simulink model "Islanding_case"  (R2024b)
settings: Solver=ode3  StartTime=0.0  StopTime=2.8  FixedStep=Ts  RelTol=1e-3  EnableMultiTasking=on
InitFcn:
  | Ts=100e-6;
  | Ts_Control=100e-6;
  | Ts_Power=100e-6;
  | tvv=0.1;
  | tr=1;
  | RelayEnableTime=1;
  | En_MC=1;
  | 
  | % ================= CHOOSE THE CASE HERE ==================
  | CaseNo    = 1;      % 1 = grid connected   2 = islanding   3 = fault during islanding
  | FaultType = 'none';   % 'none'  'LG'  'LL'  'LLG'  'LLL'  'LLLG'   (not used in case 2)
  | Qmismatch = 0;      % extra capacitive reactive power (% of 1.5 MW per load); try 1 in case 2 to see the inverter trip
  | % =========================================================
  | 
  | % ---- settings derived from the case (no need to edit)
  | switch CaseNo
  |     case 1, Tisland = 100; Pmismatch = 50; Tf = 2.0;   % grid + PV supply the load, fault at 2.0 s
  |     case 2, Tisland = 2.0; Pmismatch = 0;  Tf = 100;   % breakers open at 2.0 s, no fault
  |     case 3, Tisland = 2.0; Pmismatch = 0;  Tf = 2.3;   % breakers open at 2.0 s, fault at 2.3 s
  |     otherwise, error('CaseNo must be 1, 2 or 3');
  | end
  | FaultDur = 0.1;     % fault duration (s)
  | Tf_LG   = 100; Tf_LL = 100; Tf_LLG = 100; Tf_LLL = 100; Tf_LLLG = 100;   % 100 = never
  | switch upper(FaultType)
  |     case 'LG',   Tf_LG   = Tf;
  |     case 'LL',   Tf_LL   = Tf;
  |     case 'LLG',  Tf_LLG  = Tf;
  |     case 'LLL',  Tf_LLL  = Tf;
  |     case 'LLLG', Tf_LLLG = Tf;
  |     case 'NONE'
  |     otherwise, error('FaultType must be none, LG, LL, LLG, LLL or LLLG');
  | end
undefined symbols (not defined in the file or in its folder): DiscIntNeverNeededParam, Finit, Newton, Raphson, Tisland
libraries: simulink x33, spsOnDelayLib x17, powerlib_extras x11, eeGeneralControl x9, spsThreePhaseFaultLib x6, slpidlib x6, spsThreePhaseVIMeasurementLib x4, spsSampleandHoldLib x4, spsAlphaBetaZerotodq0Lib x4, spsThreePhaseSourceLib x4, spsThreePhaseBreakerLib x3, simulink_extras x3
(part 2 of 4)

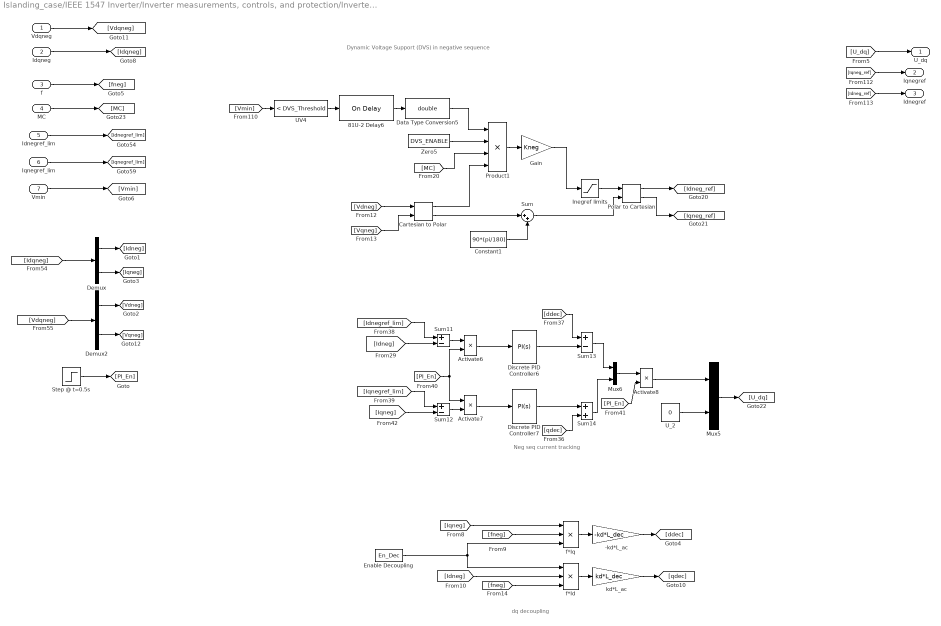
== system Islanding_case/IEEE 1547 Inverter/Inverter measurements, controls, and protection/Inverter control in negative sequence ==
  note: dq decoupling
  note: Neg seq current tracking
  note: Dynamic Voltage Support (DVS) in negative sequence
  Vdqneg : Inport
  Idqneg : Inport  Port=2
  f : Inport  Port=3
  MC : Inport  Port=4
  Idnegref_lim : Inport  Port=5
  Iqnegref_lim : Inport  Port=6
  Vmin : Inport  Port=7
  -kd*L_ac : Gain  Gain=-kd*L_dec  SaturateOnIntegerOverflow=on  OutDataTypeStr=Inherit: Same as input  ParamDataTypeStr=Inherit: Same as input
  81U-2 Delay6 : spsOnDelayLib/On Delay  DelayType=Off delay  delay=0.016  ic=0  Ts=0
  Activate6 : Product  OutDataTypeStr=double  RndMeth=Zero
  Activate7 : Product  OutDataTypeStr=double  RndMeth=Zero
  Activate8 : Product  OutDataTypeStr=double  RndMeth=Zero
  Cartesian to Polar : simulink_extras/Transformations/Cartesian to Polar
  Constant1 : Constant  Value=90*(pi/180)
  Data Type Conversion5 : DataTypeConversion  OutDataTypeStr=double  SaturateOnIntegerOverflow=off  RndMeth=Floor
  Demux : Demux  Outputs=2
  Demux2 : Demux  Outputs=2
  Discrete PID Controller6 : slpidlib/PID Controller  Controller=PI  Form=Parallel  TimeDomain=Continuous-time  UseExternalTs=off  SampleTime=-1  IntegratorMethod=Forward Euler  FilterMethod=Forward Euler  ControllerParametersSource=internal  P=Kpi  I=Kii  UseKiTs=off  D=0  UseExternalDerivativeSource=off  N=100  UseFilter=on  TunerSelectOption=Transfer Function Based (PID Tuner App)  InitialConditionSource=internal  InitialConditionForIntegrator=0  InitialConditionForFilter=0  DifferentiatorICPrevScaledInput=0  ExternalReset=none  TrackingMode=off  Kt=1  LimitOutput=on  SatLimitsSource=internal  UpperSaturationLimit=1  LowerSaturationLimit=-1  LinearizeAsGain=off  AntiWindupMode=none  Kb=1  LimitIntegrator=off  UpperIntegratorSaturationLimit=inf  LowerIntegratorSaturationLimit=-inf  POutMin=[]  POutMax=[]  IOutMin=[]  IOutMax=[]  DOutMin=[]  DOutMax=[]  NOutMin=[]  NOutMax=[]  SumOutMin=[]  SumOutMax=[]  SaturationOutMin=[]  SaturationOutMax=[]  PParamMin=[]  PParamMax=[]  IParamMin=[]  IParamMax=[]  DParamMin=[]  DParamMax=[]  NParamMin=[]  NParamMax=[]  KbParamMin=[]  KbParamMax=[]  KtParamMin=[]  KtParamMax=[]  KbOutMin=[]  KbOutMax=[]  KtOutMin=[]  KtOutMax=[]  IntegratorOutMin=[]  IntegratorOutMax=[]  FilterOutMin=[]  FilterOutMax=[]  SumI1OutMin=[]  SumI1OutMax=[]  SumI2OutMin=[]  SumI2OutMax=[]  SumI3OutMin=[]  SumI3OutMax=[]  SumI4OutMin=[]  SumI4OutMax=[]  SumDOutMin=[]  SumDOutMax=[]  DifferentiatorOutMin=[]  DifferentiatorOutMax=[]  FilterDiffOutCoefMin=[]  FilterDiffOutCoefMax=[]  ReciprocalOutMin=[]  ReciprocalOutMax=[]  SumDenOutMin=[]  SumDenOutMax=[]  SumNumOutMin=[]  SumNumOutMax=[]  DivideOutMin=[]  DivideOutMax=[]  UdiffTsProdOutMin=[]  UdiffTsProdOutMax=[]  NTsProdOutMin=[]  NTsProdOutMax=[]  UintegralTsProdOutMin=[]  UintegralTsProdOutMax=[]  UngainTsProdOutMin=[]  UngainTsProdOutMax=[]  ClampingZeroOutDataTypeStr=Inherit: Inherit via back propagation  ClampingZeroOutMin=[]  ClampingZeroOutMax=[]  FilterDenConstantOutDataTypeStr=Inherit: Inherit via back propagation  FilterDenConstantOutMin=[]  FilterDenConstantOutMax=[]  PCopyOutDataTypeStr=Inherit: Inherit via back propagation  PCopyOutMin=[]  PCopyOutMax=[]  NCopyOutDataTypeStr=Inherit: Inherit via back propagation  NCopyOutMin=[]  NCopyOutMax=[]  IntegratorContinuousStateAttributes=''  IntegratorStateMustResolveToSignalObject=off  IntegratorRTWStateStorageClass=Auto  FilterContinuousStateAttributes=''  FilterStateMustResolveToSignalObject=off  FilterRTWStateStorageClass=Auto  ParallelPVariant=InternalParameters  IdealPVariant=Disabled  IVariant=InternalParameters  DVariant=Disabled  IntegratorVariant=Continuous  SatVariant=Enabled  AWVariant=Passthrough  PCopyVariant=Disabled  TRVariant=Disabled  FdbkBlocksVariant=Forward  IdealPFdbkVariant=Disabled  SatFdbkVariant=Disabled  DerivativeFilterVariant=Disabled  NVariant=Disabled  NCopyVariant=Disabled_SignalSpec  FilterICVariant=Disabled  IntegratorICVariant=InternalICs  ExternalResetVariant=Disabled  TRSumVariant=Passthrough  SumFdbkVariant=Disabled  SumVariant=Sum_PI  TsampFilterVariant=InternalTs  TsampNgainVariant=Passthrough  TsampIntegralVariant=Disabled_SignalSpec  ExternalSaturationOutDataTypeStr=Inherit: Same as second input  DerivativeSourceVariant=Disabled  PreIntVariant=InternalPreInt
  Discrete PID Controller7 : slpidlib/PID Controller  Controller=PI  Form=Parallel  TimeDomain=Continuous-time  UseExternalTs=off  SampleTime=-1  IntegratorMethod=Forward Euler  FilterMethod=Forward Euler  ControllerParametersSource=internal  P=Kpi  I=Kii  UseKiTs=off  D=0  UseExternalDerivativeSource=off  N=100  UseFilter=on  TunerSelectOption=Transfer Function Based (PID Tuner App)  InitialConditionSource=internal  InitialConditionForIntegrator=0  InitialConditionForFilter=0  DifferentiatorICPrevScaledInput=0  ExternalReset=none  TrackingMode=off  Kt=1  LimitOutput=on  SatLimitsSource=internal  UpperSaturationLimit=1  LowerSaturationLimit=-1  LinearizeAsGain=off  AntiWindupMode=none  Kb=1  LimitIntegrator=off  UpperIntegratorSaturationLimit=inf  LowerIntegratorSaturationLimit=-inf  POutMin=[]  POutMax=[]  IOutMin=[]  IOutMax=[]  DOutMin=[]  DOutMax=[]  NOutMin=[]  NOutMax=[]  SumOutMin=[]  SumOutMax=[]  SaturationOutMin=[]  SaturationOutMax=[]  PParamMin=[]  PParamMax=[]  IParamMin=[]  IParamMax=[]  DParamMin=[]  DParamMax=[]  NParamMin=[]  NParamMax=[]  KbParamMin=[]  KbParamMax=[]  KtParamMin=[]  KtParamMax=[]  KbOutMin=[]  KbOutMax=[]  KtOutMin=[]  KtOutMax=[]  IntegratorOutMin=[]  IntegratorOutMax=[]  FilterOutMin=[]  FilterOutMax=[]  SumI1OutMin=[]  SumI1OutMax=[]  SumI2OutMin=[]  SumI2OutMax=[]  SumI3OutMin=[]  SumI3OutMax=[]  SumI4OutMin=[]  SumI4OutMax=[]  SumDOutMin=[]  SumDOutMax=[]  DifferentiatorOutMin=[]  DifferentiatorOutMax=[]  FilterDiffOutCoefMin=[]  FilterDiffOutCoefMax=[]  ReciprocalOutMin=[]  ReciprocalOutMax=[]  SumDenOutMin=[]  SumDenOutMax=[]  SumNumOutMin=[]  SumNumOutMax=[]  DivideOutMin=[]  DivideOutMax=[]  UdiffTsProdOutMin=[]  UdiffTsProdOutMax=[]  NTsProdOutMin=[]  NTsProdOutMax=[]  UintegralTsProdOutMin=[]  UintegralTsProdOutMax=[]  UngainTsProdOutMin=[]  UngainTsProdOutMax=[]  ClampingZeroOutDataTypeStr=Inherit: Inherit via back propagation  ClampingZeroOutMin=[]  ClampingZeroOutMax=[]  FilterDenConstantOutDataTypeStr=Inherit: Inherit via back propagation  FilterDenConstantOutMin=[]  FilterDenConstantOutMax=[]  PCopyOutDataTypeStr=Inherit: Inherit via back propagation  PCopyOutMin=[]  PCopyOutMax=[]  NCopyOutDataTypeStr=Inherit: Inherit via back propagation  NCopyOutMin=[]  NCopyOutMax=[]  IntegratorContinuousStateAttributes=''  IntegratorStateMustResolveToSignalObject=off  IntegratorRTWStateStorageClass=Auto  FilterContinuousStateAttributes=''  FilterStateMustResolveToSignalObject=off  FilterRTWStateStorageClass=Auto  ParallelPVariant=InternalParameters  IdealPVariant=Disabled  IVariant=InternalParameters  DVariant=Disabled  IntegratorVariant=Continuous  SatVariant=Enabled  AWVariant=Passthrough  PCopyVariant=Disabled  TRVariant=Disabled  FdbkBlocksVariant=Forward  IdealPFdbkVariant=Disabled  SatFdbkVariant=Disabled  DerivativeFilterVariant=Disabled  NVariant=Disabled  NCopyVariant=Disabled_SignalSpec  FilterICVariant=Disabled  IntegratorICVariant=InternalICs  ExternalResetVariant=Disabled  TRSumVariant=Passthrough  SumFdbkVariant=Disabled  SumVariant=Sum_PI  TsampFilterVariant=InternalTs  TsampNgainVariant=Passthrough  TsampIntegralVariant=Disabled_SignalSpec  ExternalSaturationOutDataTypeStr=Inherit: Same as second input  DerivativeSourceVariant=Disabled  PreIntVariant=InternalPreInt
  Enable Decoupling : Constant  Value=En_Dec
  Gain : Gain  Gain=Kneg
  Inegref limits : Saturate  UpperLimit=Imax  LowerLimit=0
  Mux5 : Mux  Inputs=2
  Mux6 : Mux  Inputs=2
  Polar to Cartesian : simulink_extras/Transformations/Polar to Cartesian
  Product1 : Product  Inputs=4  RndMeth=Zero
  "Step @ t=0.5s " : Step  Time=0.05  SampleTime=0
  Sum : Sum  Inputs=|++
  Sum11 : Sum  Inputs=+-
  Sum12 : Sum  Inputs=+-
  Sum13 : Sum  Inputs=+-
  Sum14 : Sum
  UV4 : simulink/Logic and Bit Operations/Compare To Constant  relop=<  const=DVS_Threshold  OutDataTypeStr=boolean  ZeroCross=off
  U_2 : Constant  Value=0
  Zero5 : Constant  Value=DVS_ENABLE
  f*Id : Product  Inputs=3  OutDataTypeStr=double  RndMeth=Zero
  f*Iq : Product  Inputs=3  OutDataTypeStr=double  RndMeth=Zero
  kd*L_ac : Gain  Gain=kd*L_dec  SaturateOnIntegerOverflow=on  OutDataTypeStr=Inherit: Same as input  ParamDataTypeStr=Inherit: Same as input
  U_dq : Outport  VectorParamsAs1DForOutWhenUnconnected=off
  Iqnegref : Outport  Port=2  VectorParamsAs1DForOutWhenUnconnected=off
  Idnegref : Outport  Port=3  VectorParamsAs1DForOutWhenUnconnected=off
  wires:
  Gain/1 -> Inegref limits/1
  Product1/1 -> Gain/1
  Data Type Conversion5/1 -> Product1/1
  [MC] -> Product1/3
  Zero5/1 -> Product1/2
  Cartesian to Polar/1 -> Product1/4
  UV4/1 -> 81U-2 Delay6/1
  [Vmin] -> UV4/1
  81U-2 Delay6/1 -> Data Type Conversion5/1
  Vmin/1 -> [Vmin]
  Inegref limits/1 -> Polar to Cartesian/1
  Idnegref_lim/1 -> [Idnegref_lim]
  [Idneg_ref] -> Idnegref/1
  Iqnegref_lim/1 -> [Iqnegref_lim]
  [Iqneg_ref] -> Iqnegref/1
  MC/1 -> [MC]
  Discrete PID Controller6/1 -> Sum13/2
  Activate6/1 -> Discrete PID Controller6/1
  Sum11/1 -> Activate6/1
  [Iqnegref_lim] -> Sum12/1
  Sum14/1 -> Mux6/2
  Sum13/1 -> Mux6/1
  Activate7/1 -> Discrete PID Controller7/1
  [Iqneg] -> Sum12/2
  [PI_En] -> Activate8/2
  Activate8/1 -> Mux5/1
  Mux5/1 -> [U_dq]
  Mux6/1 -> Activate8/1
  [qdec] -> Sum14/2
  Discrete PID Controller7/1 -> Sum14/1
  U_2/1 -> Mux5/2
  [Idnegref_lim] -> Sum11/1
  [Idneg] -> Sum11/2
  Sum12/1 -> Activate7/2
  [PI_En] -> Activate6/2, Activate7/1
  [ddec] -> Sum13/1
  "Step @ t=0.5s "/1 -> [PI_En]
  f/1 -> [fneg]
  [fneg] -> f*Id/3
  Enable Decoupling/1 -> f*Iq/3, f*Id/1
  f*Id/1 -> kd*L_ac/1
  -kd*L_ac/1 -> [ddec]
  [Idneg] -> f*Id/2
  kd*L_ac/1 -> [qdec]
  [fneg] -> f*Iq/2
  [Iqneg] -> f*Iq/1
  f*Iq/1 -> -kd*L_ac/1
  Demux/2 -> [Iqneg]
  [Vdqneg] -> Demux2/1
  Demux2/2 -> [Vqneg]
  Demux2/1 -> [Vdneg]
  Demux/1 -> [Idneg]
  [Idqneg] -> Demux/1
  Polar to Cartesian/2 -> [Iqneg_ref]
  Polar to Cartesian/1 -> [Idneg_ref]
  Sum/1 -> Polar to Cartesian/2
  Cartesian to Polar/2 -> Sum/1
  [Vqneg] -> Cartesian to Polar/2
  [Vdneg] -> Cartesian to Polar/1
  Constant1/1 -> Sum/2
  [U_dq] -> U_dq/1
  Idqneg/1 -> [Idqneg]
  Vdqneg/1 -> [Vdqneg]

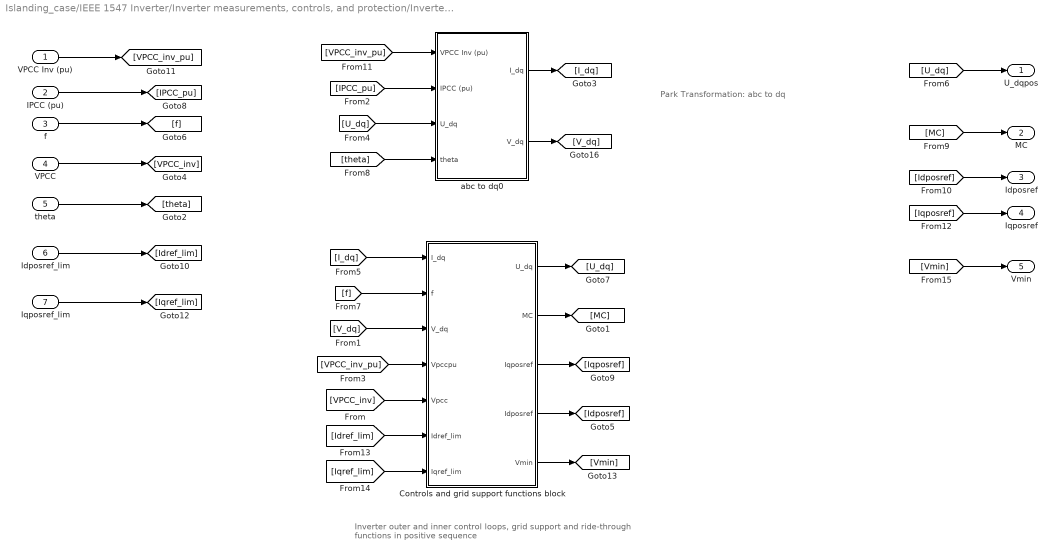
== system Islanding_case/IEEE 1547 Inverter/Inverter measurements, controls, and protection/Inverter control in positive sequence ==
  note: Park Transformation: abc to dq
  note: Inverter outer and inner control loops, grid support and ride-through functions in positive sequence
  VPCC Inv (pu) : Inport
  IPCC (pu) : Inport  Port=2
  f : Inport  Port=3
  VPCC : Inport  Port=4
  theta : Inport  Port=5
  Idposref_lim : Inport  Port=6
  Iqposref_lim : Inport  Port=7
  Controls and grid support functions block : Subsystem  mask(DQ Regulator){Kpi=0.6, Kii=100, Kpp=0.05, Kip=20, kd=1, L_dec=0.1417, En_Dec=0}
      mask prompts: Kpi "Current Proportional Gain (Kpi)"; Kii "Current Integral Gain (Kii)"; Kpp "Power Proportional Gain (Kpp)"; Kip "Power Integral Gain (Kip)"; kd "Decoupling Gain (kd)"; L_dec "Decoupling inductance (L_dec)"; En_Dec "Enable Decoupling (En_Dec) (1-Enabled, 0-Disabled)"
      mask help:
      | This block contains PI controllers that track the reference signal Idq_ref.
      | The PI gains are masked along with the decoupling gain kd.  DC voltage tracking
      | might also be implemented in this block.
      mask init:
      | if(En_Dec ~=1) %anything but 1 disables the decoupling
      |     En_Dec = 0;
      | end
      mask DialogControl Desc Prompt: ToolBarParametersMenu
  "abc to dq0 " : Subsystem
  U_dqpos : Outport  VectorParamsAs1DForOutWhenUnconnected=off
  MC : Outport  Port=2  VectorParamsAs1DForOutWhenUnconnected=off
  Idposref : Outport  Port=3  VectorParamsAs1DForOutWhenUnconnected=off
  Iqposref : Outport  Port=4  VectorParamsAs1DForOutWhenUnconnected=off
  Vmin : Outport  Port=5  VectorParamsAs1DForOutWhenUnconnected=off
  wires:
  [Vmin] -> Vmin/1
  Controls and grid support functions block/5(Vmin) -> [Vmin]
  Controls and grid support functions block/4(Idposref) -> [Idposref]
  Controls and grid support functions block/3(Iqposref) -> [Iqposref]
  Iqposref_lim/1 -> [Iqref_lim]
  Idposref_lim/1 -> [Idref_lim]
  [Iqref_lim] -> Controls and grid support functions block/7(Iqref_lim)
  [Idref_lim] -> Controls and grid support functions block/6(Idref_lim)
  [Iqposref] -> Iqposref/1
  [Idposref] -> Idposref/1
  [MC] -> MC/1
  Controls and grid support functions block/2(MC) -> [MC]
  [theta] -> "abc to dq0 "/4(theta)
  theta/1 -> [theta]
  [U_dq] -> U_dqpos/1
  VPCC/1 -> [VPCC_inv]
  [VPCC_inv] -> Controls and grid support functions block/5(Vpcc)
  [VPCC_inv_pu] -> Controls and grid support functions block/4(Vpccpu)
  [VPCC_inv_pu] -> "abc to dq0 "/1(VPCC Inv (pu))
  [IPCC_pu] -> "abc to dq0 "/2(IPCC (pu))
  [V_dq] -> Controls and grid support functions block/3(V_dq)
  VPCC Inv (pu)/1 -> [VPCC_inv_pu]
  [f] -> Controls and grid support functions block/2(f)
  Controls and grid support functions block/1(U_dq) -> [U_dq]
  [I_dq] -> Controls and grid support functions block/1(I_dq)
  "abc to dq0 "/1(I_dq) -> [I_dq]
  [U_dq] -> "abc to dq0 "/3(U_dq)
  IPCC (pu)/1 -> [IPCC_pu]
  f/1 -> [f]
  "abc to dq0 "/2(V_dq) -> [V_dq]

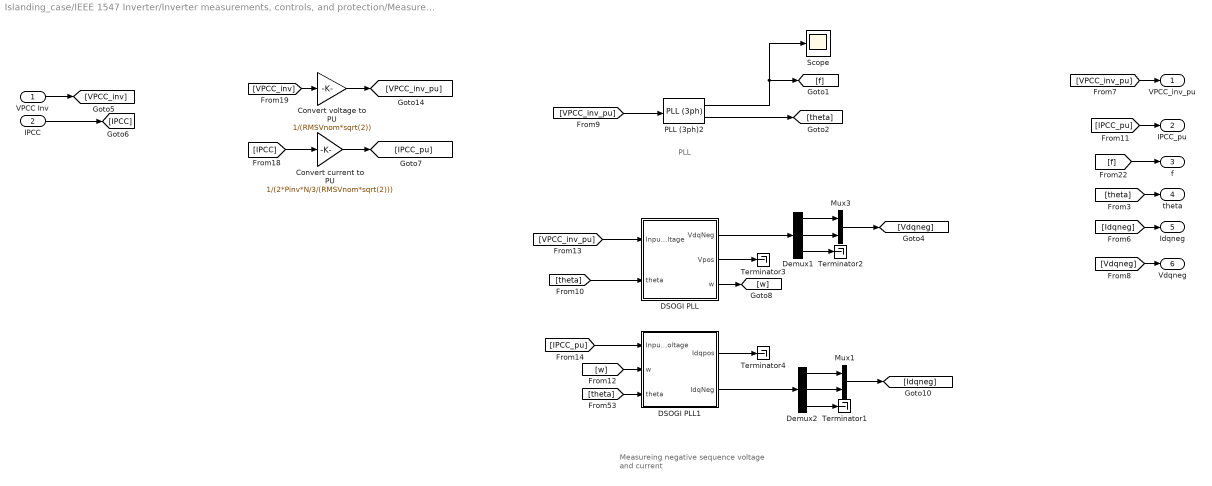
== system Islanding_case/IEEE 1547 Inverter/Inverter measurements, controls, and protection/Measurements ==
  note: Measureing negative sequence voltage and current
  note: PLL
  VPCC Inv : Inport
  IPCC : Inport  Port=2
  Convert current to PU : Gain  Gain=1/(2*Pinv*N/3/(RMSVnom*sqrt(2)))  SaturateOnIntegerOverflow=on  OutDataTypeStr=Inherit: Same as input  ParamDataTypeStr=Inherit: Same as input
  Convert voltage to PU : Gain  Gain=1/(RMSVnom*sqrt(2))  SaturateOnIntegerOverflow=on  OutDataTypeStr=Inherit: Same as input  ParamDataTypeStr=Inherit: Same as input
  DSOGI PLL : Subsystem
  DSOGI PLL1 : Subsystem
  Demux1 : Demux  Outputs=3
  Demux2 : Demux  Outputs=3
  Mux1 : Mux  Inputs=2
  Mux3 : Mux  Inputs=2
  PLL (3ph)2 : spsPLL3phLib/PLL (3ph)  Fmin=48  Par_Init=[0, NomFreq]  ParK=[180/2.5 3200/1.25 0.25]  TcD=1e-4  MaxRateChangeFreq=24  FilterCutOffFreq=200  Ts=0  AGC=off
  Scope : Scope
  Terminator{1..4} (4 alike) : Terminator
  VPCC_inv_pu : Outport  VectorParamsAs1DForOutWhenUnconnected=off
  IPCC_pu : Outport  Port=2  VectorParamsAs1DForOutWhenUnconnected=off
  f : Outport  Port=3  VectorParamsAs1DForOutWhenUnconnected=off
  theta : Outport  Port=4  VectorParamsAs1DForOutWhenUnconnected=off
  Idqneg : Outport  Port=5  VectorParamsAs1DForOutWhenUnconnected=off
  Vdqneg : Outport  Port=6  VectorParamsAs1DForOutWhenUnconnected=off
  wires:
  DSOGI PLL1/1(Idqpos) -> Terminator4/1
  Mux1/1 -> [Idqneg]
  Demux2/1 -> Mux1/1
  Demux2/3 -> Terminator1/1
  DSOGI PLL1/2(IdqNeg) -> Demux2/1
  Demux2/2 -> Mux1/2
  DSOGI PLL/2(Vpos) -> Terminator3/1
  DSOGI PLL/3(w) -> [w]
  Mux3/1 -> [Vdqneg]
  Demux1/3 -> Terminator2/1
  Demux1/2 -> Mux3/2
  Demux1/1 -> Mux3/1
  DSOGI PLL/1(VdqNeg) -> Demux1/1
  [theta] -> DSOGI PLL1/3(theta)
  [IPCC_pu] -> DSOGI PLL1/1(InputVoltage)
  [theta] -> DSOGI PLL/2(theta)
  [w] -> DSOGI PLL1/2("w ")
  [VPCC_inv_pu] -> DSOGI PLL/1(InputVoltage)
  PLL (3ph)2/1 -> [f], Scope/1
  PLL (3ph)2/2 -> [theta]
  [VPCC_inv_pu] -> PLL (3ph)2/1
  [Vdqneg] -> Vdqneg/1
  [Idqneg] -> Idqneg/1
  [theta] -> theta/1
  [VPCC_inv] -> Convert voltage to PU/1
  [IPCC_pu] -> IPCC_pu/1
  [VPCC_inv_pu] -> VPCC_inv_pu/1
  Convert current to PU/1 -> [IPCC_pu]
  Convert voltage to PU/1 -> [VPCC_inv_pu]
  [f] -> f/1
  [IPCC] -> Convert current to PU/1
  VPCC Inv/1 -> [VPCC_inv]
  IPCC/1 -> [IPCC]

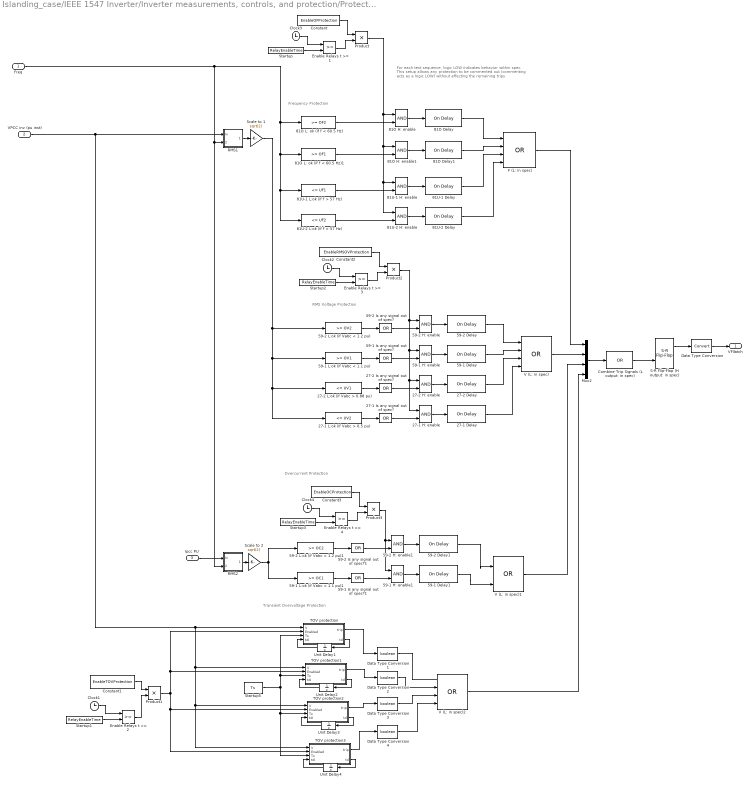
== system Islanding_case/IEEE 1547 Inverter/Inverter measurements, controls, and protection/Protection  ==
  note: Transient Overvoltage Protection
  note: Overcurrent Protection
  note: For each test sequence, logic LOW indicates behavior within spec. This setup allows any protection to be commented out (commenting acts as a logic LOW) without affecting the remaining trips.
  note: RMS Voltage Protection
  note: Frequency Protection
  Freq : Inport
  VPCC inv (pu inst) : Inport  Port=2
  Ipcc PU : Inport  Port=3
  27-1 Delay : spsOnDelayLib/On Delay  DelayType=On delay  delay=UV2_time  ic=0  Ts=0
  27-1 H: enable : Logic  IconShape=distinctive  AllPortsSameDT=off  OutDataTypeStr=boolean
  27-1 Is any signal out of spec? : Logic  Operator=OR  Inputs=1  IconShape=distinctive  AllPortsSameDT=off  OutDataTypeStr=boolean
  27-1 L:ok (if Vabc > 0.5 pu) : simulink/Logic and Bit Operations/Compare To Constant  relop=<=  const=UV2  OutDataTypeStr=boolean  ZeroCross=off
  27-2 Delay : spsOnDelayLib/On Delay  DelayType=On delay  delay=UV1_time  ic=0  Ts=0
  27-2 H: enable : Logic  IconShape=distinctive  AllPortsSameDT=off  OutDataTypeStr=boolean
  27-2 Is any signal out of spec? : Logic  Operator=OR  Inputs=1  IconShape=distinctive  AllPortsSameDT=off  OutDataTypeStr=boolean
  27-2 L:ok (if Vabc > 0.88 pu) : simulink/Logic and Bit Operations/Compare To Constant  relop=<=  const=UV1  OutDataTypeStr=boolean  ZeroCross=off
  59-1 Delay : spsOnDelayLib/On Delay  DelayType=On delay  delay=OV1_time  ic=0  Ts=0
  59-1 Delay1 : spsOnDelayLib/On Delay  DelayType=On delay  delay=OC1_time  ic=0  Ts=0
  59-1 H: enable : Logic  IconShape=distinctive  AllPortsSameDT=off  OutDataTypeStr=boolean
  59-1 H: enable1 : Logic  IconShape=distinctive  AllPortsSameDT=off  OutDataTypeStr=boolean
  59-1 Is any signal out of spec? : Logic  Operator=OR  Inputs=1  IconShape=distinctive  AllPortsSameDT=off  OutDataTypeStr=boolean
  59-1 Is any signal out of spec?1 : Logic  Operator=OR  Inputs=1  IconShape=distinctive  AllPortsSameDT=off  OutDataTypeStr=boolean
  59-1 L:ok (if Vabc < 1.1 pu) : simulink/Logic and Bit Operations/Compare To Constant  relop=>=  const=OV1  OutDataTypeStr=boolean  ZeroCross=off
  59-1 L:ok (if Vabc < 1.1 pu)1 : simulink/Logic and Bit Operations/Compare To Constant  relop=>=  const=OC1  OutDataTypeStr=boolean  ZeroCross=off
  59-2 Delay : spsOnDelayLib/On Delay  DelayType=On delay  delay=OV2_time  ic=0  Ts=0
  59-2 Delay1 : spsOnDelayLib/On Delay  DelayType=On delay  delay=OC2_time  ic=0  Ts=0
  59-2 H: enable : Logic  IconShape=distinctive  AllPortsSameDT=off  OutDataTypeStr=boolean
  59-2 H: enable1 : Logic  IconShape=distinctive  AllPortsSameDT=off  OutDataTypeStr=boolean
  59-2 Is any signal out of spec? : Logic  Operator=OR  Inputs=1  IconShape=distinctive  AllPortsSameDT=off  OutDataTypeStr=boolean
  59-2 Is any signal out of spec?1 : Logic  Operator=OR  Inputs=1  IconShape=distinctive  AllPortsSameDT=off  OutDataTypeStr=boolean
  59-2 L:ok (if Vabc < 1.2 pu) : simulink/Logic and Bit Operations/Compare To Constant  relop=>=  const=OV2  OutDataTypeStr=boolean  ZeroCross=off
  59-2 L:ok (if Vabc < 1.2 pu)1 : simulink/Logic and Bit Operations/Compare To Constant  relop=>=  const=OC2  OutDataTypeStr=boolean  ZeroCross=off
  81O Delay : spsOnDelayLib/On Delay  DelayType=On delay  delay=OF2_time  ic=0  Ts=0
  81O Delay1 : spsOnDelayLib/On Delay  DelayType=On delay  delay=OF1_time  ic=0  Ts=0
  81O H: enable : Logic  IconShape=distinctive  AllPortsSameDT=off  OutDataTypeStr=boolean
  81O H: enable1 : Logic  IconShape=distinctive  AllPortsSameDT=off  OutDataTypeStr=boolean
  81O L: ok (if f < 60.5 Hz) : simulink/Logic and Bit Operations/Compare To Constant  relop=>=  const=OF2  OutDataTypeStr=boolean  ZeroCross=off
  81O L: ok (if f < 60.5 Hz)1 : simulink/Logic and Bit Operations/Compare To Constant  relop=>=  const=OF1  OutDataTypeStr=boolean  ZeroCross=off
  81U-1 Delay : spsOnDelayLib/On Delay  DelayType=On delay  delay=UF1_time  ic=0  Ts=0
  81U-1 H: enable : Logic  IconShape=distinctive  AllPortsSameDT=off  OutDataTypeStr=boolean
  81U-1 L:ok (if f > 57 Hz) : simulink/Logic and Bit Operations/Compare To Constant  relop=<=  const=UF1  OutDataTypeStr=boolean  ZeroCross=off
  81U-2 Delay : spsOnDelayLib/On Delay  DelayType=On delay  delay=UF2_time  ic=0  Ts=0
  81U-2 H: enable : Logic  IconShape=distinctive  AllPortsSameDT=off  OutDataTypeStr=boolean
  81U-2 L:ok (if f > 57 Hz) : simulink/Logic and Bit Operations/Compare To Constant  relop=<=  const=UF2  OutDataTypeStr=boolean  ZeroCross=off
  Clock{1..4} (4 alike) : Clock
  Combine Trip Signals (L output: in spec) : Logic  Operator=OR  Inputs=1  IconShape=distinctive  AllPortsSameDT=off  OutDataTypeStr=boolean
  Constant : Constant  Value=EnableOFProtection  SampleTime=-1
  Constant1 : Constant  Value=EnableTOVProtection  SampleTime=-1
  Constant2 : Constant  Value=EnableRMSOVProtection  SampleTime=-1
  Constant3 : Constant  Value=EnableOCProtection  SampleTime=-1
  Data Type Conversion : DataTypeConversion  SaturateOnIntegerOverflow=off  RndMeth=Floor
  Data Type Conversion{1..4} (4 alike) : DataTypeConversion  OutDataTypeStr=boolean  SaturateOnIntegerOverflow=off  RndMeth=Floor
  Enable Relays t >= {1..4} (4 alike) : RelationalOperator  OutDataTypeStr=boolean  InputSameDT=off
  F (L: in spec) : Logic  Operator=OR  Inputs=4  IconShape=distinctive  AllPortsSameDT=off  OutDataTypeStr=boolean
  Mux2 : Mux
  Product{,1..3} (4 alike) : Product
  RMS1 : Subsystem  AncestorBlock=|  DialogController=POWERSYS.PowerSysDialog  mask(Discrete RMS value){Mag_Init=0, Ts=Ts}
      | powerlib_extras/Discrete
      | Measurements/Discrete 
      | RMS value
      mask prompts: Mag_Init "Initial magnitude of input:"; Ts "Sample time:"
      mask help:
      | Measure the true root mean square (RMS) value of a signal.
      |
      | To measure the RMS value of the fundamental component, use instead the Discrete Fourier block and divide its output by sqrt(2).
      mask init:
      | power_initmask();
      mask Help: web(psbhelp)
      mask Display: disp('RMS\n(discrete)')
  RMS2 : Subsystem  AncestorBlock=|  DialogController=POWERSYS.PowerSysDialog  mask(Discrete RMS value){Mag_Init=0, Ts=Ts}
      | powerlib_extras/Discrete
      | Measurements/Discrete 
      | RMS value
      mask prompts: Mag_Init "Initial magnitude of input:"; Ts "Sample time:"
      mask help:
      | Measure the true root mean square (RMS) value of a signal.
      |
      | To measure the RMS value of the fundamental component, use instead the Discrete Fourier block and divide its output by sqrt(2).
      mask init:
      | power_initmask();
      mask Help: web(psbhelp)
      mask Display: disp('RMS\n(discrete)')
  S-R Flip-Flop (H output: in spec) : simulink_extras/Flip Flops/S-R Flip-Flop  initial_condition=1
  Scale to 1 : Gain  Gain=sqrt(2)  SaturateOnIntegerOverflow=on  OutDataTypeStr=Inherit: Same as input  ParamDataTypeStr=Inherit: Same as input
  Scale to 2 : Gain  Gain=sqrt(2)  SaturateOnIntegerOverflow=on  OutDataTypeStr=Inherit: Same as input  ParamDataTypeStr=Inherit: Same as input
  Startup{,1..3} (4 alike) : Constant  Value=RelayEnableTime
  Startup5 : Constant  Value=Ts
  TOV protection : MATLAB Function  TreatAsAtomicUnit=on
  TOV protection1 : MATLAB Function  TreatAsAtomicUnit=on
  TOV protection2 : MATLAB Function  TreatAsAtomicUnit=on
  TOV protection3 : MATLAB Function  TreatAsAtomicUnit=on
  Unit Delay{1..4} (4 alike) : UnitDelay  SampleTime=-1  HasFrameUpgradeWarning=on
  V (L: in spec) : Logic  Operator=OR  Inputs=4  IconShape=distinctive  AllPortsSameDT=off  OutDataTypeStr=boolean
  V (L: in spec)1 : Logic  Operator=OR  IconShape=distinctive  AllPortsSameDT=off  OutDataTypeStr=boolean
  V (L: in spec)2 : Logic  Operator=OR  Inputs=4  IconShape=distinctive  AllPortsSameDT=off  OutDataTypeStr=boolean
  VFIlatch : Outport  VectorParamsAs1DForOutWhenUnconnected=off
  wires:
  Startup5/1 -> TOV protection/3(Ts), TOV protection1/3(Ts), TOV protection3/3(Ts), TOV protection2/3(Ts)
  Product3/1 -> 59-2 H: enable1/1, 59-1 H: enable1/1
  Enable Relays t >= 4/1 -> Product3/2
  Startup3/1 -> Enable Relays t >= 4/2
  Clock4/1 -> Enable Relays t >= 4/1
  Constant3/1 -> Product3/1
  Product2/1 -> 59-2 H: enable/1, 59-1 H: enable/1, 27-2 H: enable/1, 27-1 H: enable/1
  Enable Relays t >= 3/1 -> Product2/2
  Startup2/1 -> Enable Relays t >= 3/2
  Clock2/1 -> Enable Relays t >= 3/1
  Constant2/1 -> Product2/1
  Enable Relays t >= 2/1 -> Product1/2
  Startup1/1 -> Enable Relays t >= 2/2
  Constant1/1 -> Product1/1
  Clock1/1 -> Enable Relays t >= 2/1
  Enable Relays t >= 1/1 -> Product/2
  Startup/1 -> Enable Relays t >= 1/2
  Clock3/1 -> Enable Relays t >= 1/1
  Constant/1 -> Product/1
  TOV protection/1(trip) -> Data Type Conversion1/1
  Data Type Conversion3/1 -> V (L: in spec)2/3
  TOV protection2/1(trip) -> Data Type Conversion3/1
  TOV protection/2(td) -> Unit Delay1/1
  TOV protection3/1(trip) -> Data Type Conversion4/1
  Unit Delay1/1 -> TOV protection/4(tdi)
  Unit Delay4/1 -> TOV protection3/4(tdi)
  Unit Delay2/1 -> TOV protection1/4(tdi)
  TOV protection2/2(td) -> Unit Delay3/1
  TOV protection1/2(td) -> Unit Delay2/1
  TOV protection3/2(td) -> Unit Delay4/1
  Product/1 -> 81O H: enable/1, 81U-2 H: enable/1, 81U-1 H: enable/1, 81O H: enable1/1
  TOV protection1/1(trip) -> Data Type Conversion2/1
  Data Type Conversion2/1 -> V (L: in spec)2/2
  Data Type Conversion4/1 -> V (L: in spec)2/4
  Product1/1 -> TOV protection1/2(Enabled), TOV protection/2(Enabled), TOV protection2/2(Enabled), TOV protection3/2(Enabled)
  Data Type Conversion1/1 -> V (L: in spec)2/1
  VPCC inv (pu inst)/1 -> TOV protection1/1(V), TOV protection3/1(V), TOV protection2/1(V), TOV protection/1(V), RMS1/1(In)
  Unit Delay3/1 -> TOV protection2/4(tdi)
  V (L: in spec)2/1 -> Mux2/4
  RMS2/1(RMS) -> Scale to 2/1
  V (L: in spec)1/1 -> Mux2/3
  59-1 Delay1/1 -> V (L: in spec)1/2
  59-1 L:ok (if Vabc < 1.1 pu)1/1 -> 59-1 Is any signal out of spec?1/1
  59-2 Is any signal out of spec?1/1 -> 59-2 H: enable1/2
  59-2 Delay1/1 -> V (L: in spec)1/1
  59-2 H: enable1/1 -> 59-2 Delay1/1
  59-2 L:ok (if Vabc < 1.2 pu)1/1 -> 59-2 Is any signal out of spec?1/1
  59-1 Is any signal out of spec?1/1 -> 59-1 H: enable1/2
  59-1 H: enable1/1 -> 59-1 Delay1/1
  Ipcc PU/1 -> RMS2/1(In)
  Scale to 2/1 -> 59-1 L:ok (if Vabc < 1.1 pu)1/1, 59-2 L:ok (if Vabc < 1.2 pu)1/1
  Freq/1 -> RMS1/2(Freq), RMS2/2(Freq), 81U-1 L:ok (if f > 57 Hz)/1, 81U-2 L:ok (if f > 57 Hz)/1, 81O L: ok (if f < 60.5 Hz)1/1, 81O L: ok (if f < 60.5 Hz)/1
  S-R Flip-Flop (H output: in spec)/1 -> Data Type Conversion/1
  27-1 Delay/1 -> V (L: in spec)/4
  27-2 Delay/1 -> V (L: in spec)/3
  59-1 Delay/1 -> V (L: in spec)/2
  59-2 Delay/1 -> V (L: in spec)/1
  81U-2 Delay/1 -> F (L: in spec)/4
  81U-1 Delay/1 -> F (L: in spec)/3
  81O Delay1/1 -> F (L: in spec)/2
  81O H: enable1/1 -> 81O Delay1/1
  81O L: ok (if f < 60.5 Hz)1/1 -> 81O H: enable1/2
  Scale to 1/1 -> 59-2 L:ok (if Vabc < 1.2 pu)/1, 27-2 L:ok (if Vabc > 0.88 pu)/1, 27-1 L:ok (if Vabc > 0.5 pu)/1, 59-1 L:ok (if Vabc < 1.1 pu)/1
  Mux2/1 -> Combine Trip Signals (L output: in spec)/1
  Data Type Conversion/1 -> VFIlatch/1
  Combine Trip Signals (L output: in spec)/1 -> S-R Flip-Flop (H output: in spec)/2
  81U-2 L:ok (if f > 57 Hz)/1 -> 81U-2 H: enable/2
  81U-2 H: enable/1 -> 81U-2 Delay/1
  59-2 Is any signal out of spec?/1 -> 59-2 H: enable/2
  59-2 L:ok (if Vabc < 1.2 pu)/1 -> 59-2 Is any signal out of spec?/1
  59-2 H: enable/1 -> 59-2 Delay/1
  81U-1 L:ok (if f > 57 Hz)/1 -> 81U-1 H: enable/2
  81U-1 H: enable/1 -> 81U-1 Delay/1
  RMS1/1(RMS) -> Scale to 1/1
  81O L: ok (if f < 60.5 Hz)/1 -> 81O H: enable/2
  81O H: enable/1 -> 81O Delay/1
  59-1 Is any signal out of spec?/1 -> 59-1 H: enable/2
  59-1 L:ok (if Vabc < 1.1 pu)/1 -> 59-1 Is any signal out of spec?/1
  59-1 H: enable/1 -> 59-1 Delay/1
  27-2 Is any signal out of spec?/1 -> 27-2 H: enable/2
  27-2 L:ok (if Vabc > 0.88 pu)/1 -> 27-2 Is any signal out of spec?/1
  27-2 H: enable/1 -> 27-2 Delay/1
  27-1 Is any signal out of spec?/1 -> 27-1 H: enable/2
  27-1 L:ok (if Vabc > 0.5 pu)/1 -> 27-1 Is any signal out of spec?/1
  27-1 H: enable/1 -> 27-1 Delay/1
  81O Delay/1 -> F (L: in spec)/1
  V (L: in spec)/1 -> Mux2/2
  F (L: in spec)/1 -> Mux2/1

== system Islanding_case/IEEE 1547 Inverter/Inverter measurements, controls, and protection/abc to dq0 and dq0 to abc negative1 ==
  U_dq+ : Inport
  U_dq- : Inport  Port=2
  theta : Inport  Port=3
  Gain : Gain  Gain=-1
  Sum : Sum  Inputs=|++
  dq0 to abc : spsdq0toabcLib/dq0 to abc  Alignment=90 degrees behind phase A axis
  dq0 to abc1 : spsdq0toabcLib/dq0 to abc  Alignment=90 degrees behind phase A axis
  Uref : Outport  VectorParamsAs1DForOutWhenUnconnected=off
  wires:
  dq0 to abc1/1 -> [UrefN]
  dq0 to abc/1 -> [UrefP]
  [theta] -> dq0 to abc/2
  [U_dqpos] -> dq0 to abc/1
  Sum/1 -> [Uref]
  [UrefN] -> Sum/2
  [UrefP] -> Sum/1
  Gain/1 -> dq0 to abc1/2
  [theta] -> Gain/1
  [U_dqneg] -> dq0 to abc1/1
  theta/1 -> [theta]
  U_dq-/1 -> [U_dqneg]
  [Uref] -> Uref/1
  U_dq+/1 -> [U_dqpos]
